simulink model "opamp"  (Simulink 7.0)
settings: Solver=ode45  StartTime=0.0  StopTime=10.0  RelTol=1e-3
settings Model: Creator=107108103  LastModifiedBy=107108103

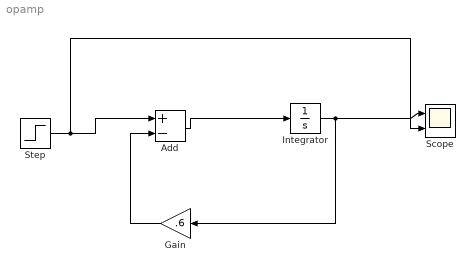
== system opamp ==
  Add : Sum  Inputs=+-  OutDataType=sfix(16)  OutScaling=2^-10
  Gain : Gain  Orientation=left  Gain=.6  ParameterDataType=sfix(16)  ParameterScaling=2^0  OutDataType=sfix(16)  OutScaling=2^0
  Integrator : Integrator  LimitOutput=on  UpperSaturationLimit=15  LowerSaturationLimit=-15
  Scope : Scope  NumInputPorts=2
      settings: YMin=-5~-5  YMax=5~5
  Step : Step  SampleTime=0
  wires:
  Step/1 -> Add/1, Scope/2
  Gain/1 -> Add/2
  Add/1 -> Integrator/1
  Integrator/1 -> Gain/1, Scope/1
